simulink model "test5_orig"  (R2017b)
settings: Solver=VariableStepAuto  StartTime=0.0  StopTime=10.0  RelTol=1e-3
settings Model: Creator=monika  LastModifiedBy=monika

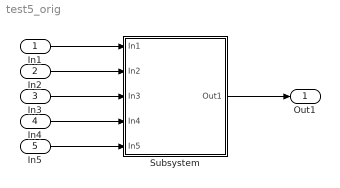
== system test5_orig ==
  In1 : Inport
  In2 : Inport  Port=2
  In3 : Inport  Port=3
  In4 : Inport  Port=4
  In5 : Inport  Port=5
  Subsystem : Subsystem
  Out1 : Outport
  wires:
  In2/1 -> Subsystem/2(In2)
  In1/1 -> Subsystem/1(In1)
  In3/1 -> Subsystem/3(In3)
  In4/1 -> Subsystem/4(In4)
  Subsystem/1(Out1) -> Out1/1
  In5/1 -> Subsystem/5(In5)

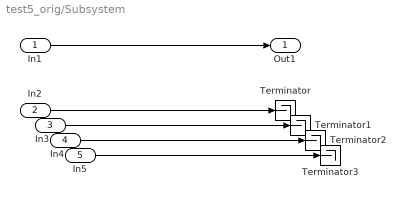
== system test5_orig/Subsystem ==
  In1 : Inport
  In2 : Inport  Port=2
  In3 : Inport  Port=3
  In4 : Inport  Port=4
  In5 : Inport  Port=5
  Terminator{,1..3} (4 alike) : Terminator
  Out1 : Outport
  wires:
  In1/1 -> Out1/1
  In2/1 -> Terminator/1
  In3/1 -> Terminator1/1
  In4/1 -> Terminator2/1
  In5/1 -> Terminator3/1
